simulink model "tmp"  (Simulink 8.5)
settings: Solver=ode45  StartTime=0.0  StopTime=10.0  RelTol=1e-3
undefined symbols (not defined in the file or in its folder): Kd, Ki, Kp, lambda
libraries: nintblocks x2
settings Model: Creator=felipe  LastModifiedBy=felipe
settings DataIOCC: SignalLoggingSaveFormat=Dataset
settings OptimizationCC: ExpressionDepthLimit=128
settings DebuggingCC: UnderspecifiedInitializationDetection=Simplified  MergeDetectMultiDrivingBlocksExec=error  FcnCallInpInsideContextMsg=EnableAllAsError  StateNameClashWarn=none
settings GRTTargetCC: CombineOutputUpdateFcns=on  GRTInterface=off

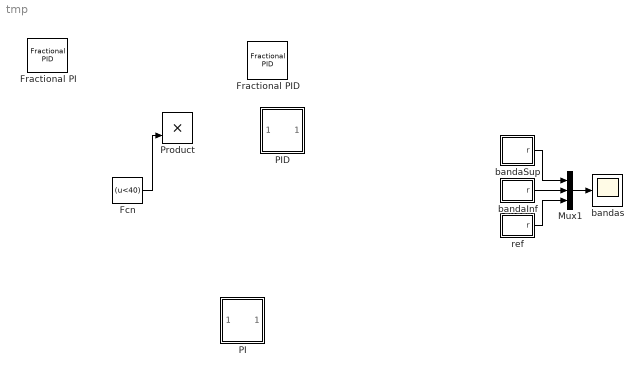
== system tmp ==
  Fcn : Fcn  Expr=(u<40)
  Fractional PI : nintblocks/Fractional PID  kp=Kp  kd=Kd  vd=mu  ki=Ki  vi=-lambda  bandwidth=[0.01 100]  n=100  form1=crone  exp1=mcltime  decomp1=frac
  Fractional PID : nintblocks/Fractional PID  kp=Kp  kd=Kd  vd=mu  ki=Ki  vi=-lambda  bandwidth=[0.01 100]  n=100  form1=crone  exp1=mcltime  decomp1=frac
  Mux1 : Mux  Inputs=3
  PI : Subsystem
  PID : Subsystem
  Product : Product
  bandaInf : Subsystem
  bandaSup : Subsystem
  bandas : Scope
      settings: TimeRange=971.6614906832298  YMin=14.5  YMax=22.5  SaveName=bandas
  ref : Subsystem
  wires:
  Mux1/1 -> bandas/1
  bandaSup/1(r) -> Mux1/1
  bandaInf/1(r) -> Mux1/2
  ref/1(r) -> Mux1/3
  ? -> Product/1
  Fcn/1 -> Product/2

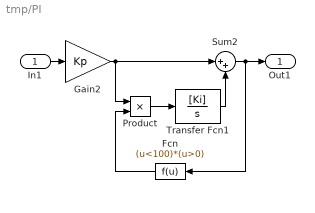
== system tmp/PI ==
  In1 : Inport
  Fcn : Fcn  Expr=(u<100)*(u>0)
  Gain2 : Gain  Gain=Kp
  Product : Product  RndMeth=Zero
  Sum2 : Sum  Inputs=|++
  Transfer Fcn1 : TransferFcn  Numerator=[Ki]  Denominator=[1 0]
  Out1 : Outport
  wires:
  Gain2/1 -> Sum2/1, Product/1
  Sum2/1 -> Fcn/1, Out1/1
  Transfer Fcn1/1 -> Sum2/2
  Product/1 -> Transfer Fcn1/1
  Fcn/1 -> Product/2
  In1/1 -> Gain2/1

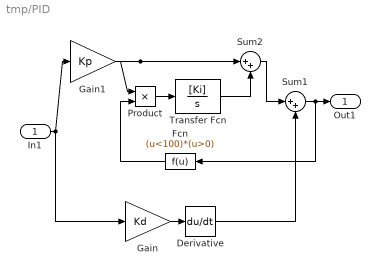
== system tmp/PID ==
  In1 : Inport
  Derivative : Derivative
  Fcn : Fcn  Expr=(u<100)*(u>0)
  Gain : Gain  Gain=Kd
  Gain1 : Gain  Gain=Kp
  Product : Product  RndMeth=Zero
  Sum1 : Sum  Inputs=|++
  Sum2 : Sum  Inputs=|++
  Transfer Fcn : TransferFcn  Numerator=[Ki]  Denominator=[1 0]
  Out1 : Outport
  wires:
  Gain/1 -> Derivative/1
  Gain1/1 -> Sum2/1, Product/1
  Sum2/1 -> Sum1/1
  Transfer Fcn/1 -> Sum2/2
  Product/1 -> Transfer Fcn/1
  Fcn/1 -> Product/2
  In1/1 -> Gain/1, Gain1/1
  Sum1/1 -> Out1/1, Fcn/1
  Derivative/1 -> Sum1/2

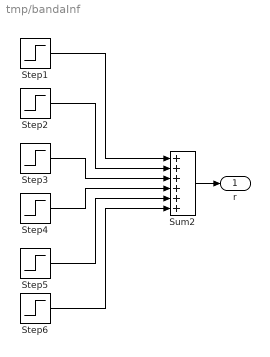
== system tmp/bandaInf ==
  Step1 : Step  Time=400  Before=22.5*0.98  After=22.5*0.98  SampleTime=0
  Step2 : Step  Time=401  After=15*0.98
  Step3 : Step  Time=801  After=15*0.98
  Step4 : Step  Time=1201  After=-15*0.98
  Step5 : Step  Time=1601  After=-15*0.98
  Step6 : Step  Time=2001  After=-7.5*0.98
  Sum2 : Sum  Inputs=++++++
  r : Outport
  wires:
  Sum2/1 -> r/1
  Step1/1 -> Sum2/1
  Step2/1 -> Sum2/2
  Step5/1 -> Sum2/5
  Step6/1 -> Sum2/6
  Step3/1 -> Sum2/3
  Step4/1 -> Sum2/4

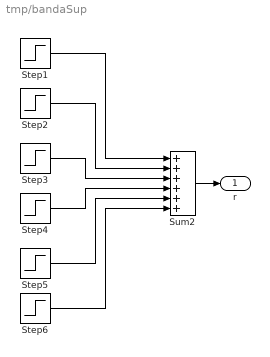
== system tmp/bandaSup ==
  Step1 : Step  Time=400  Before=22.5*(1.02)  After=22.5*(1.02)  SampleTime=0
  Step2 : Step  Time=401  After=15*(1.02)
  Step3 : Step  Time=801  After=15*(1.02)
  Step4 : Step  Time=1201  After=-15*(1.02)
  Step5 : Step  Time=1601  After=-15*(1.02)
  Step6 : Step  Time=2001  After=-7.5*(1.02)
  Sum2 : Sum  Inputs=++++++
  r : Outport
  wires:
  Sum2/1 -> r/1
  Step1/1 -> Sum2/1
  Step2/1 -> Sum2/2
  Step5/1 -> Sum2/5
  Step6/1 -> Sum2/6
  Step3/1 -> Sum2/3
  Step4/1 -> Sum2/4

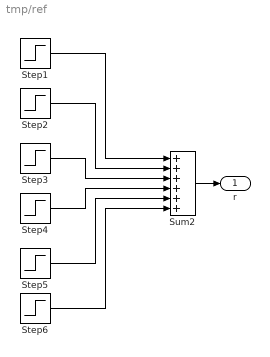
== system tmp/ref ==
  Step1 : Step  Time=400  Before=22.5  After=22.5  SampleTime=0
  Step2 : Step  Time=401  After=15
  Step3 : Step  Time=801  After=15
  Step4 : Step  Time=1201  After=-15
  Step5 : Step  Time=1601  After=-15
  Step6 : Step  Time=2001  After=-7.5
  Sum2 : Sum  Inputs=++++++
  r : Outport
  wires:
  Sum2/1 -> r/1
  Step1/1 -> Sum2/1
  Step2/1 -> Sum2/2
  Step5/1 -> Sum2/5
  Step6/1 -> Sum2/6
  Step3/1 -> Sum2/3
  Step4/1 -> Sum2/4
